simulink model "champer"  (R2019a)
settings: Solver=VariableStepAuto  StartTime=0.0  StopTime=10.0  RelTol=1e-3
settings Model: Creator=Raouf  LastModifiedBy=Raouf

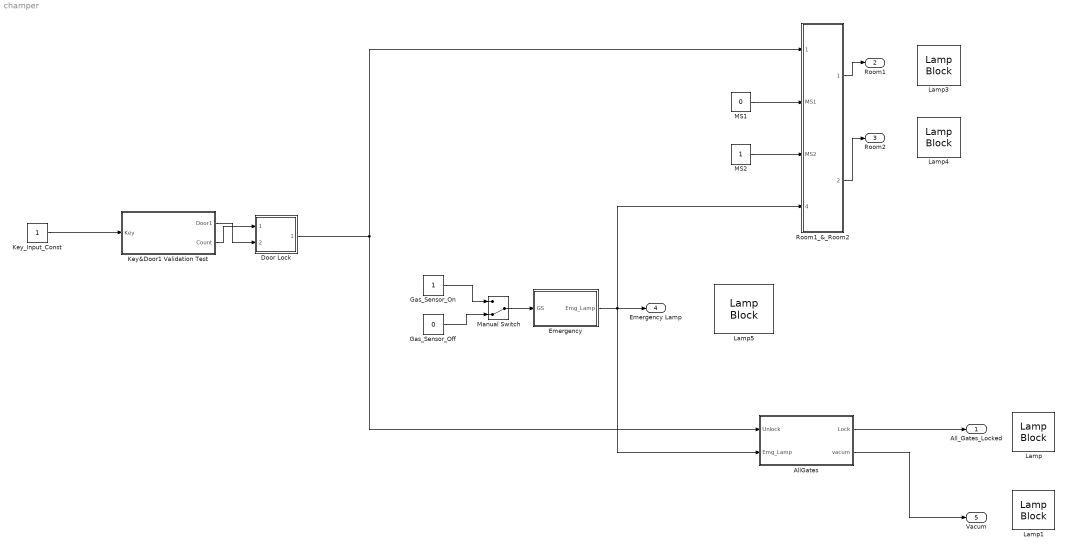
== system champer ==
  AllGates : Stateflow chart  BlockKeywords=__PRM__SERIALIZED__DATA__:Stateflow Chart,Stateflow Diagram  TreatAsAtomicUnit=on
  Door Lock : Stateflow chart  BlockKeywords=__PRM__SERIALIZED__DATA__:Stateflow Chart,Stateflow Diagram  TreatAsAtomicUnit=on
  Emergency : Stateflow chart  BlockKeywords=__PRM__SERIALIZED__DATA__:Stateflow Chart,Stateflow Diagram  TreatAsAtomicUnit=on
  Gas_Sensor_Off : Constant  Value=0  OutDataTypeStr=boolean
  Gas_Sensor_On : Constant  OutDataTypeStr=boolean
  Key&Door1 Validation Test : Stateflow chart  BlockKeywords=__PRM__SERIALIZED__DATA__:Stateflow Chart,Stateflow Diagram  TreatAsAtomicUnit=on
  Key_Input_Const : Constant  OutDataTypeStr=uint16
  Lamp{,1,3..5} (5 alike) : LampBlock
  MS1 : Constant  Value=0  OutDataTypeStr=boolean
  MS2 : Constant  OutDataTypeStr=boolean
  Manual Switch : ManualSwitch  CurrentSetting=0
  Room1_&_Room2 : Stateflow chart  BlockKeywords=__PRM__SERIALIZED__DATA__:Stateflow Chart,Stateflow Diagram  TreatAsAtomicUnit=on
  All_Gates_Locked : Outport
  Room1 : Outport  Port=2
  Room2 : Outport  Port=3
  Emergency Lamp : Outport  Port=4
  Vacum : Outport  Port=5
  wires:
  Key&Door1 Validation Test/1(Door1) -> Door Lock/2(Door1)
  Key&Door1 Validation Test/2(Count) -> Door Lock/1(Count)
  Door Lock/1(Unlock) -> AllGates/1(Unlock), Room1_&_Room2/1(Unlock)
  AllGates/1(Lock) -> All_Gates_Locked/1
  Key_Input_Const/1 -> Key&Door1 Validation Test/1(Key)
  Room1_&_Room2/1(Lamp1) -> Room1/1
  Room1_&_Room2/2(Lamp2) -> Room2/1
  MS2/1 -> Room1_&_Room2/3(MS2)
  MS1/1 -> Room1_&_Room2/2(MS1)
  Emergency/1(Emg_Lamp) -> Room1_&_Room2/4(Emg_Lamp), Emergency Lamp/1, AllGates/2(Emg_Lamp)
  Manual Switch/1 -> Emergency/1(GS)
  Gas_Sensor_On/1 -> Manual Switch/1
  Gas_Sensor_Off/1 -> Manual Switch/2
  AllGates/2(vacum) -> Vacum/1

== stateflow chart champer/Door Lock ==
  (default) -> (junction 11) : % DoorLock
  (junction 11) -> (junction 12) [order 1] : [(Count < 3)&&(Door1 == 1)]
  (junction 11) -> (junction 13) [order 2]
  (junction 12) -> (junction 17) : {Unlock = 1;}
  (junction 13) -> (junction 14) [order 1] : [(Count < 3)&&(Door1 == 0)]
  (junction 13) -> (junction 15) [order 2] : {Unlock = -1;}
  (junction 14) -> (junction 16) : {Unlock = 0;}
  (junction 16) -> (junction 15)
  (junction 17) -> (junction 16)
  (junction 15) -> (junction 18)
  data: Count input uint8; Door1 input boolean; Unlock output int8

== stateflow chart champer/AllGates ==
  state Normal_Behavior
    entry:
    vacum = 0;
  state Close_Gates
    entry:
    vacum = 0;
    during:
    vacum = 1;
  (default) -> (junction 7) : % GatesLock
  (junction 7) -> (junction 8) [order 1] : [Unlock == -1 && Emg_Lamp == 0]
  (junction 7) -> (junction 9) [order 2] : {Lock = 0;}
  (junction 8) -> (junction 10) : {Lock = 1;}
  (junction 10) -> (junction 9)
  (junction 9) -> (junction 31)
  (junction 31) -> (junction 32) [order 1] : [Emg_Lamp == 1]
  (junction 32) -> (junction 52)
  (junction 31) -> Normal_Behavior [order 2]
  (junction 53) -> (junction 51) [order 1] : [x < 5]
  (junction 51) -> (junction 54) : {/* delay(1000) */;}
  (junction 52) -> (junction 53) : {x = 0;}
  (junction 54) -> (junction 53) : {x = x+1;}
  (junction 53) -> (junction 55) [order 2]
  (junction 55) -> Close_Gates
  data: Unlock input int8; Lock output boolean; Emg_Lamp input boolean; vacum output boolean; x local double

== stateflow chart champer/Key&Door1 Validation Test ==
  (default) -> (junction 9) : % Key&Door=>1
  (junction 9) -> (junction 10) [order 1] : [Key == 1]
  (junction 10) -> (junction 37) : {Door1 = 1;
      |  Count = 0;}
  (junction 9) -> (junction 22) [order 2] : {Door1 = 0;
      |  Count = 1;}
  (junction 22) -> (junction 23) [order 1] : [Key == 1]
  (junction 23) -> (junction 37) : {Door1 = 1;
      | Count = 0;}
  (junction 22) -> (junction 34) [order 2] : {Door1 = 0;
      |  Count = Count + 1;}
  (junction 34) -> (junction 36) [order 1] : [Key == 1]
  (junction 36) -> (junction 37) : {Door1 = 1;
      | Count = 0;}
  (junction 34) -> (junction 37) [order 2] : {Door1 = 0;
      |  Count = Count + 1;}
  data: Key input uint16; Door1 output boolean; Count output uint8

== stateflow chart champer/Room1_&_Room2 ==
  state TurnOn_Lamp1
    en:
    Lamp1 = 1;
  state TurnOff_Lamp1
    en:
    Lamp1 = 0;
  state TurnOn_Lamp2
    en:
    Lamp2 = 1;
  state TurnOff_Lamp2
    en:
    Lamp2 = 0;
  (default) -> (junction 20) : /* Unlocked Gates Room1*/
  (junction 20) -> (junction 21) [order 1] : [Unlock == 1 && Emg_Lamp == 0 && MS1 == 1 && MS2 == 0]
  (junction 20) -> TurnOff_Lamp1 [order 2]
  (junction 21) -> TurnOn_Lamp1 : {Lamp2 = 0;}
  TurnOff_Lamp1 -> (junction 53)
  (junction 53) -> (junction 54) [order 1] : [Unlock == 1 && Emg_Lamp == 0 && MS2 == 1 && MS1 == 0]
  (junction 53) -> TurnOff_Lamp2 [order 2]
  (junction 54) -> TurnOn_Lamp2 : {Lamp1 = 0;}
  data: Unlock input int8; Lamp1 output boolean; Lamp2 output boolean; MS1 input boolean; MS2 input boolean; Emg_Lamp input boolean

== stateflow chart champer/Emergency ==
  state Emg_Lamp
    en:
    Emg_Lamp = 0;
  state Emg_Lamp_
    en:
    Emg_Lamp = 1;
  (default) -> (junction 7) : % Emergency
  (junction 7) -> (junction 8) [order 1] : [GS == 1]
  (junction 7) -> Emg_Lamp [order 2]
  (junction 8) -> Emg_Lamp_
  data: GS input boolean; Emg_Lamp output boolean
